simulink model "ExCount_naive_model_R2012b"  (Simulink 8.0)
settings: Solver=ode45  StartTime=0.0  StopTime=100e-6  RelTol=1e-3
values from neighbouring files (symbols this model uses):
  fsig = 13.0e3    (= 13000)    [ExCount.m]
  M = OSR    (= 16)    [ExCount.m]
  OSR = 16    [ExCount.m]
  tclk = Ts    (= 6.25e-07)    [ExCount.m]
  Ts = 1/fs    (= 6.25e-07)    [ExCount.m]
  vfs = vref*2    (= 1.8)    [ExCount.m]
  vin_amp = 10.^(vin_amp_dB/20)*vref    [ExCount.m]
  vref = 0.9    [ExCount.m]
libraries: dspsigops x2
settings Model: Creator=chench  LastModifiedBy=benve
settings OptimizationCC: InitFltsAndDblsToZero=on
settings DebuggingCC: SaveWithParameterizedLinksMsg=none  SignalResolutionControl=TryResolveAllWithWarning  MultiTaskDSMMsg=warning  MultiTaskCondExecSysMsg=none  FcnCallInpInsideContextMsg=EnableAllAsWarning  FrameProcessingCompatibilityMsg=error
settings CodeAppCC: CustomSymbolStrType=$N$R$M_T
settings GRTTargetCC: TargetFcnLib=ansi_tfl_tmw.mat  CodeReplacementLibrary=C89/C90 (ANSI)  CombineOutputUpdateFcns=off  GRTInterface=on

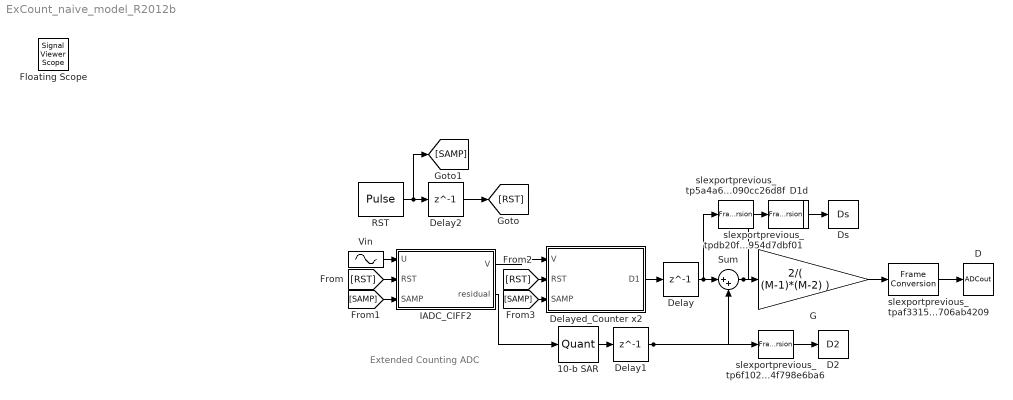
== system ExCount_naive_model_R2012b ==
  note: Extended Counting ADC
  10-b SAR : Quantizer  QuantizationInterval=vfs/1024  LinearizeAsGain=off
  D : ToWorkspace  VariableName=ADCout  SampleTime=-1
  D1d : ToWorkspace  VariableName=D1d  SampleTime=-1
  D2 : ToWorkspace  VariableName=D2  SampleTime=-1
  Delay : Delay  DelayLength=1  InitialCondition=0  SampleTime=Ts*OSR
  Delay1 : Delay  DelayLength=1  InitialCondition=0  SampleTime=Ts*OSR
  Delay2 : Delay  DelayLength=1  InitialCondition=0
  Delayed_Counter x2 : Subsystem
  Ds : ToWorkspace  VariableName=Ds  SampleTime=-1
  G : Gain  Gain=2/( (M-1)*(M-2) )
  IADC_CIFF2 : Subsystem
  RST : DiscretePulseGenerator  Period=OSR  SampleTime=tclk
  Sum : Sum  Inputs=|++
  Vin : Sin  Amplitude=vin_amp  Frequency=fsig*2*pi  SampleTime=tclk
  slexportprevious_tp5a4a6e99_3524_404b_8fdb_01090cc26d8f : FrameConversion  OutFrame=Sample-based
  slexportprevious_tp6f10270c_ac72_4f92_8769_a64f798e6ba6 : FrameConversion  OutFrame=Sample-based
  slexportprevious_tpaf3315f7_6e1b_448a_8f04_532706ab4209 : FrameConversion  OutFrame=Sample-based
  slexportprevious_tpdb20fef2_1793_4f8b_81d5_88954d7dbf01 : FrameConversion  OutFrame=Sample-based
  Floating Scope : SignalViewerScope  IOType=viewer  SampleTime=-1  ZoomMode=on
      settings: TimeRange=auto  TickLabels=OneTimeTick  LimitDataPoints=on  MaxDataPoints=5000  SaveToWorkspace=off  SaveName=ScopeData  YMin=-10  YMax=10  SampleInput=off  DataFormat=StructureWithTime
  wires:
  Sum/1 -> G/1, slexportprevious_tpdb20fef2_1793_4f8b_81d5_88954d7dbf01/1
  IADC_CIFF2/2(residual) -> 10-b SAR/1
  Delayed_Counter x2/1(D1) -> Delay/1
  Vin/1 -> IADC_CIFF2/1(U)
  IADC_CIFF2/1(V) -> Delayed_Counter x2/1(V)
  Delay/1 -> Sum/1, slexportprevious_tp5a4a6e99_3524_404b_8fdb_01090cc26d8f/1
  10-b SAR/1 -> Delay1/1
  Delay1/1 -> Sum/2, slexportprevious_tp6f10270c_ac72_4f92_8769_a64f798e6ba6/1
  RST/1 -> [SAMP], Delay2/1
  Delay2/1 -> [RST]
  [RST] -> IADC_CIFF2/2(RST)
  [SAMP] -> IADC_CIFF2/3(SAMP)
  [RST] -> Delayed_Counter x2/2(RST)
  [SAMP] -> Delayed_Counter x2/3(SAMP)
  G/1 -> slexportprevious_tpaf3315f7_6e1b_448a_8f04_532706ab4209/1
  slexportprevious_tpaf3315f7_6e1b_448a_8f04_532706ab4209/1 -> D/1
  slexportprevious_tp5a4a6e99_3524_404b_8fdb_01090cc26d8f/1 -> D1d/1
  slexportprevious_tp6f10270c_ac72_4f92_8769_a64f798e6ba6/1 -> D2/1
  slexportprevious_tpdb20fef2_1793_4f8b_81d5_88954d7dbf01/1 -> Ds/1

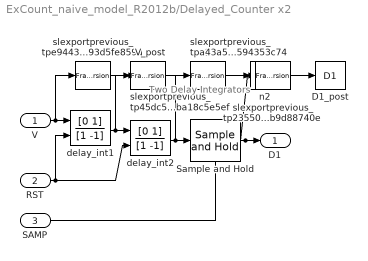
== system ExCount_naive_model_R2012b/Delayed_Counter x2 ==
  note: Two Delay Integrators
  V : Inport
  RST : Inport  Port=2
  SAMP : Inport  Port=3
  D1_post : ToWorkspace  VariableName=D1  SampleTime=-1
  Sample and Hold : dspsigops/Sample and Hold  trig=Rising edge  initCond=0  latchinput=off
  V_post : ToWorkspace  VariableName=V  SampleTime=-1
  delay_int1 : DiscreteFilter  Numerator=[0 1]  Denominator=[1 -1]  ExternalReset=Rising
      settings: InputPortMap=u0,r7
  delay_int2 : DiscreteFilter  Numerator=[0 1]  Denominator=[1 -1]  ExternalReset=Rising
      settings: InputPortMap=u0,r7
  n1 : ToWorkspace  VariableName=n1  SampleTime=-1
  n2 : ToWorkspace  VariableName=n2  SampleTime=-1
  slexportprevious_tp235505b7_d880_4864_8977_523b9d88740e : FrameConversion  OutFrame=Sample-based
  slexportprevious_tp45dc5b6e_0c89_4657_9d22_12ba18c5e5ef : FrameConversion  OutFrame=Sample-based
  slexportprevious_tpa43a5871_c6f5_408a_ab27_7e3594353c74 : FrameConversion  OutFrame=Sample-based
  slexportprevious_tpe9443a3a_c5d9_4914_896c_0c93d5fe859d : FrameConversion  OutFrame=Sample-based
  D1 : Outport
  wires:
  delay_int1/1 -> delay_int2/1, slexportprevious_tp45dc5b6e_0c89_4657_9d22_12ba18c5e5ef/1
  V/1 -> delay_int1/1, slexportprevious_tpe9443a3a_c5d9_4914_896c_0c93d5fe859d/1
  delay_int2/1 -> Sample and Hold/1, slexportprevious_tpa43a5871_c6f5_408a_ab27_7e3594353c74/1
  RST/1 -> delay_int1/2, delay_int2/2
  Sample and Hold/1 -> D1/1, slexportprevious_tp235505b7_d880_4864_8977_523b9d88740e/1
  SAMP/1 -> Sample and Hold/Trigger
  slexportprevious_tp235505b7_d880_4864_8977_523b9d88740e/1 -> D1_post/1
  slexportprevious_tpe9443a3a_c5d9_4914_896c_0c93d5fe859d/1 -> V_post/1
  slexportprevious_tp45dc5b6e_0c89_4657_9d22_12ba18c5e5ef/1 -> n1/1
  slexportprevious_tpa43a5871_c6f5_408a_ab27_7e3594353c74/1 -> n2/1

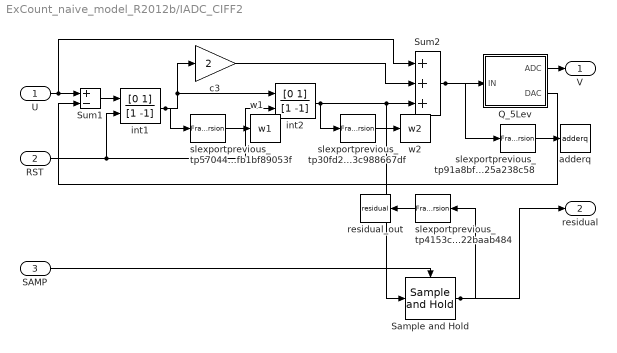
== system ExCount_naive_model_R2012b/IADC_CIFF2 ==
  U : Inport
  RST : Inport  Port=2
  SAMP : Inport  Port=3
  Q_5Lev : Subsystem
  Sample and Hold : dspsigops/Sample and Hold  trig=Rising edge  initCond=0  latchinput=off
  Sum1 : Sum  Inputs=+-  SaturateOnIntegerOverflow=on  InputSameDT=on  OutDataTypeStr=Inherit: Same as first input
  Sum2 : Sum  Inputs=+++  SaturateOnIntegerOverflow=on  InputSameDT=on  OutDataTypeStr=Inherit: Same as first input
  adderq : ToWorkspace  VariableName=adderq  SampleTime=-1
  c3 : Gain  Gain=2  SaturateOnIntegerOverflow=on  OutDataTypeStr=Inherit: Same as input  ParamDataTypeStr=Inherit: Same as input
  int1 : DiscreteFilter  Numerator=[0 1]  Denominator=[1 -1]  ExternalReset=Rising
      settings: InputPortMap=u0,r7
  int2 : DiscreteFilter  Numerator=[0 1]  Denominator=[1 -1]  ExternalReset=Rising
      settings: InputPortMap=u0,r7
  residual_out : ToWorkspace  VariableName=residual  SampleTime=-1
  slexportprevious_tp30fd26e6_8090_4d22_86ff_c53c988667df : FrameConversion  OutFrame=Sample-based
  slexportprevious_tp4153c90b_521e_4d4f_bb70_f3d22baab484 : FrameConversion  OutFrame=Sample-based
  slexportprevious_tp57044c8b_1919_4ed0_b248_ffb1bf89053f : FrameConversion  OutFrame=Sample-based
  slexportprevious_tp91a8bf55_6e9d_48cf_bc78_44d25a238c58 : FrameConversion  OutFrame=Sample-based
  w1 : ToWorkspace  VariableName=w1  SampleTime=-1
  w2 : ToWorkspace  VariableName=w2  SampleTime=-1
  V : Outport
  residual : Outport  Port=2
  wires:
  c3/1 -> Sum2/2
  Sum2/1 -> Q_5Lev/1(IN), slexportprevious_tp91a8bf55_6e9d_48cf_bc78_44d25a238c58/1
  int2/1 -> Sum2/3, Sample and Hold/1, slexportprevious_tp30fd26e6_8090_4d22_86ff_c53c988667df/1
  Q_5Lev/1(ADC) -> V/1
  Q_5Lev/2(DAC) -> Sum1/2
  Sum1/1 -> int1/1
  U/1 -> Sum2/1, Sum1/1
  RST/1 -> int2/2, int1/2
  int1/1 -> int2/1, c3/1, slexportprevious_tp57044c8b_1919_4ed0_b248_ffb1bf89053f/1
  Sample and Hold/1 -> residual/1, slexportprevious_tp4153c90b_521e_4d4f_bb70_f3d22baab484/1
  SAMP/1 -> Sample and Hold/Trigger
  slexportprevious_tp91a8bf55_6e9d_48cf_bc78_44d25a238c58/1 -> adderq/1
  slexportprevious_tp4153c90b_521e_4d4f_bb70_f3d22baab484/1 -> residual_out/1
  slexportprevious_tp57044c8b_1919_4ed0_b248_ffb1bf89053f/1 -> w1/1
  slexportprevious_tp30fd26e6_8090_4d22_86ff_c53c988667df/1 -> w2/1

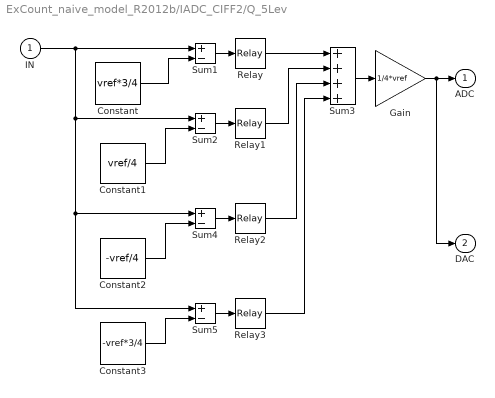
== system ExCount_naive_model_R2012b/IADC_CIFF2/Q_5Lev ==
  IN : Inport
  Constant : Constant  Value=vref*3/4
  Constant1 : Constant  Value=vref/4
  Constant2 : Constant  Value=-vref/4
  Constant3 : Constant  Value=-vref*3/4
  Gain : Gain  Gain=1/4*vref
  Relay{,1..3} (4 alike) : Relay  OffOutputValue=-1  SampleTime=tclk
  Sum{1..2,4..5} (4 alike) : Sum  Inputs=+-  SaturateOnIntegerOverflow=on  InputSameDT=on  OutDataTypeStr=Inherit: Same as first input
  Sum3 : Sum  Inputs=++++  SaturateOnIntegerOverflow=on  InputSameDT=on  OutDataTypeStr=Inherit: Same as first input
  ADC : Outport
  DAC : Outport  Port=2
  wires:
  Sum1/1 -> Relay/1
  Sum2/1 -> Relay1/1
  IN/1 -> Sum1/1, Sum2/1, Sum4/1, Sum5/1
  Constant/1 -> Sum1/2
  Constant1/1 -> Sum2/2
  Relay/1 -> Sum3/1
  Relay1/1 -> Sum3/2
  Sum3/1 -> Gain/1
  Sum4/1 -> Relay2/1
  Constant2/1 -> Sum4/2
  Relay2/1 -> Sum3/3
  Sum5/1 -> Relay3/1
  Constant3/1 -> Sum5/2
  Relay3/1 -> Sum3/4
  Gain/1 -> DAC/1, ADC/1
